simulink model "helicopter_Kalman_4dim"  (R2021b)
settings: Solver=ode45  StartTime=0.0  StopTime=T  RelTol=1e-3
InitFcn:
  | hwinit
values from neighbouring files (symbols this model uses):
  A_lin = [0, 1, 0; K1*cos(alpha_ref), -b, -2*K3*omega_ref; 0, 0, -K4 ]    [observer.m]
  B_lin = [0;0; -K4]    [observer.m]
  C = [1, 0, 0; 0, 0, 1]    [controller_LQR.m]    (also in controller_MPC.m; helicopter_EKF_code.m; observer.m; polish_MPC.m)
  h = 0.01    [Pure_Kalman_check.m]    (also in calibration.m; controller_LQR.m; controller_MPC.m; helicopter_EKF_code.m)
  K = place(A_lin, B_lin, p_new)    [helicopter_EKF_code.m]
  x_ref = sdpvar(n_x, 1)    [MPC_step.m]    (also in controller_LQR.m = [alpha_ref; alpha_dot_ref; omega_ref]/0.9; controller_MPC.m = [alpha_ref; alpha_dot_ref; omega_ref]; helicopter_EKF_code.m = [alpha_ref; alpha_dot_ref; omega_ref]; polish_MPC.m = [alpha_ref; alpha_dot_ref ; omega_ref])
undefined symbols (not defined in the file or in its folder): adingain, adinoffs, Continuous, HeliMexHandle, Time
libraries: ctrlSharedLib x1
settings Model: Creator=fkzhang  LastModifiedBy=lcaric
settings SolverCC: AlgebraicLoopSolver=TrustRegion
settings DataIOCC: LimitDataPoints=on  SaveFormat=Array  ReturnWorkspaceOutputs=off
settings OptimizationCC: BlockReduction=off  BooleanDataType=off  LifeSpan=inf
settings DebuggingCC: SaveWithParameterizedLinksMsg=none  UnderspecifiedInitializationDetection=Classic  MergeDetectMultiDrivingBlocksExec=none  SignalResolutionControl=TryResolveAllWithWarning  AllowSymbolicDim=off  SFUnexpectedBacktrackingDiag=warning  SFNoUnconditionalDefaultTransitionDiag=warning  SFExecutionAtInitializationDiag=none  SFMachineParentedDataDiag=warning  ArithmeticOperatorsInVariantConditions=warning
settings HardwareCC: ProdBitPerPointer=32  ProdBitPerSizeT=32  ProdBitPerPtrDiffT=32  ProdLargestAtomicFloat=None  ProdIntDivRoundTo=Undefined  ProdEndianess=Unspecified  ProdWordSize=32  ProdHWDeviceType=32-bit Generic  TargetUnknown=on
settings ModelReferenceCC: PropagateSignalLabelsOutOfModel=off
settings SFSimCC: SimUseLocalCustomCode=off  CustomCodeUndefinedFunction=UseInterfaceOnly
settings RTWCC: RTWUseLocalCustomCode=off
settings CodeAppCC: StateflowObjectComments=on
settings GRTTargetCC: TargetLangStandard=C89/C90 (ANSI)
settings ConfigComp: CovMetricSettings=dw  CovSaveCumulativeToWorkspaceVar=on  CovSaveSingleToWorkspaceVar=on  CovExternalEMLEnable=off  CovSFcnEnable=off

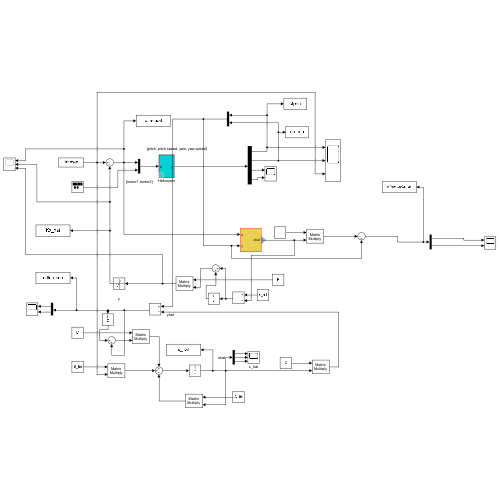
[thumbnail: Simulink's stored preview of the top-level diagram]
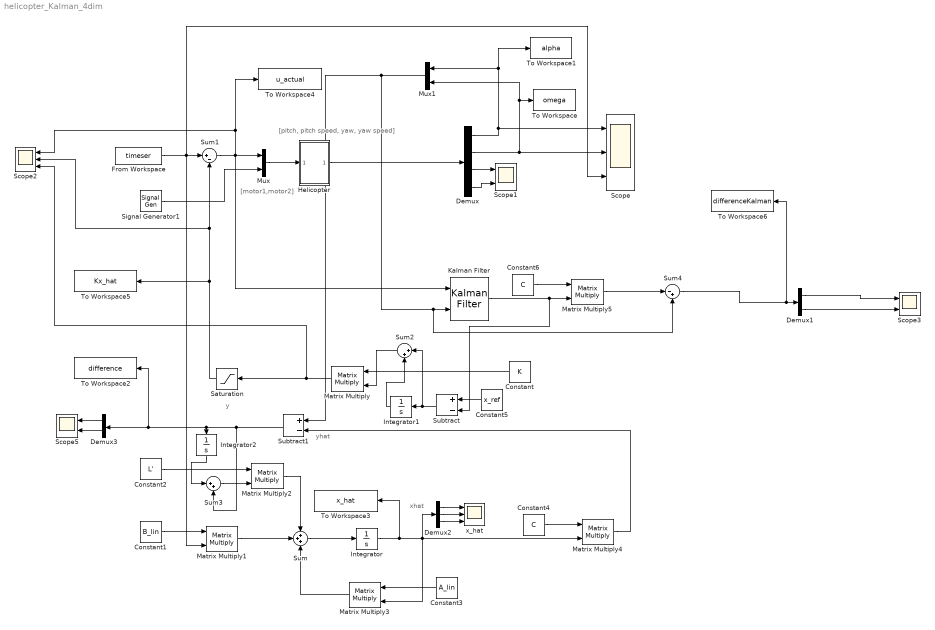
== system helicopter_Kalman_4dim ==
  note: yhat
  note: y
  note: xhat
  note: [pitch, pitch speed, yaw, yaw speed]
  note: [motor1,motor2]
  Constant : Constant  Value=K  VectorParams1D=off
  Constant1 : Constant  Value=B_lin  VectorParams1D=off
  Constant2 : Constant  Value=L'
  Constant3 : Constant  Value=A_lin
  Constant4 : Constant  Value=C
  Constant5 : Constant  Value=x_ref
  Constant6 : Constant  Value=C
  Demux : Demux
  Demux1 : Demux  Outputs=2
  Demux2 : Demux  Outputs=3
  Demux3 : Demux  Outputs=2
  From Workspace : FromWorkspace  VariableName=timeser
  Helicopter : Subsystem  mask{Ts=h}
      mask prompts: Ts "sampletime"
      mask init:
      | sf_heli_init
      mask Display:
      | port_label('input',1,'u');
      | port_label('output',1,'y');
  Integrator : Integrator
  Integrator1 : Integrator
  Integrator2 : Integrator
  Kalman Filter : ctrlSharedLib/Kalman Filter  TimeDomain=Continuous-Time  UseCurrentEstimator=on  ModelSource=LTI State-Space Variable  ModelSourceVariable=minssss  A=A_lin  B=B_lin  C=C  D=[0;0]  NumberOfStates=1  NumberOfInputs=1  NumberOfOutputs=1  InitialEstimateSource=Dialog  X0=[0;0;0;0]  P0=10  UseK=off  UseGH=off  NumberOfProcessNoiseInputs=1  G=1  TimeInvariantG=on  H=0  TimeInvariantH=on  Q=5*eye(3)  TimeInvariantQ=on  R=0.5*eye(2)  TimeInvariantR=on  N=0  TimeInvariantN=on  AddInputPort=on  AddEnablePort=off  OutputEstimatedY=off  OutputP=off  Ts=-1
  Matrix Multiply{,1..5} (6 alike) : Product  Multiplication=Matrix(*)
  Mux : Mux  Inputs=2
  Mux1 : Mux  Inputs=2
  Saturation : Saturate  UpperLimit=1  LowerLimit=-1
  Scope : Scope  NumInputPorts=3
  Scope1 : Scope  NumInputPorts=2
  Scope2 : Scope  NumInputPorts=3
  Scope3 : Scope  NumInputPorts=2
  Scope5 : Scope  NumInputPorts=2
  Signal Generator1 : SignalGenerator  WaveForm=square  Amplitude=0  Frequency=1/20
  Subtract : Sum  Inputs=+-
  Subtract1 : Sum  Inputs=+-
  Sum : Sum  Inputs=+++
  Sum1 : Sum  Inputs=|+-
  Sum2 : Sum  Inputs=|++
  Sum3 : Sum  Inputs=|++
  Sum4 : Sum  Inputs=|-+
  To Workspace : ToWorkspace  VariableName=omega  SaveFormat=Timeseries  SampleTime=-1
  To Workspace1 : ToWorkspace  VariableName=alpha  SaveFormat=Timeseries  SampleTime=-1
  To Workspace2 : ToWorkspace  VariableName=difference  SaveFormat=Timeseries  SampleTime=-1
  To Workspace3 : ToWorkspace  VariableName=x_hat  SaveFormat=Timeseries  SampleTime=-1
  To Workspace4 : ToWorkspace  VariableName=u_actual  SaveFormat=Timeseries  SampleTime=-1
  To Workspace5 : ToWorkspace  VariableName=Kx_hat  SaveFormat=Timeseries  SampleTime=-1
  To Workspace6 : ToWorkspace  VariableName=differenceKalman  SaveFormat=Timeseries  SampleTime=-1
  x_hat : Scope  NumInputPorts=3
  wires:
  Mux/1 -> Helicopter/1(In1)
  Signal Generator1/1 -> Mux/2
  Demux/2 -> Scope/2, To Workspace/1, Mux1/2
  Demux/3 -> Scope1/1
  Demux/4 -> Scope1/2
  From Workspace/1 -> Sum1/1, Matrix Multiply1/2, Scope/3
  Demux/1 -> To Workspace1/1, Mux1/1, Scope/1
  Mux1/1 -> Sum4/2, Kalman Filter/2, Subtract1/1
  Helicopter/1(Out1) -> Demux/1
  Matrix Multiply1/1 -> Sum/2
  Matrix Multiply2/1 -> Sum/1
  Sum/1 -> Integrator/1
  Matrix Multiply3/1 -> Sum/3
  Integrator/1 -> To Workspace3/1, Matrix Multiply3/2, Matrix Multiply4/2, Demux2/1
  Demux2/2 -> x_hat/2
  Demux2/3 -> x_hat/3
  Demux2/1 -> x_hat/1
  Matrix Multiply4/1 -> Subtract1/2
  Demux3/2 -> Scope5/2
  Demux3/1 -> Scope5/1
  Constant1/1 -> Matrix Multiply1/1
  Constant2/1 -> Matrix Multiply2/1
  Constant4/1 -> Matrix Multiply4/1
  Constant3/1 -> Matrix Multiply3/1
  Sum1/1 -> Kalman Filter/1, To Workspace4/1, Scope2/1, Mux/1
  Constant/1 -> Matrix Multiply/1
  Saturation/1 -> To Workspace5/1, Scope2/2, Sum1/2
  Matrix Multiply/1 -> Saturation/1, Scope2/3
  Constant5/1 -> Subtract/1
  Subtract/1 -> Sum2/1, Integrator1/1
  Integrator1/1 -> Sum2/2
  Sum2/1 -> Matrix Multiply/2
  Subtract1/1 -> To Workspace2/1, Demux3/1, Integrator2/1, Sum3/2
  Demux1/2 -> Scope3/2
  Demux1/1 -> Scope3/1
  Constant6/1 -> Matrix Multiply5/1
  Kalman Filter/1 -> Subtract/2, Matrix Multiply5/2
  Matrix Multiply5/1 -> Sum4/1
  Sum4/1 -> To Workspace6/1, Demux1/1
  Integrator2/1 -> Sum3/1
  Sum3/1 -> Matrix Multiply2/2

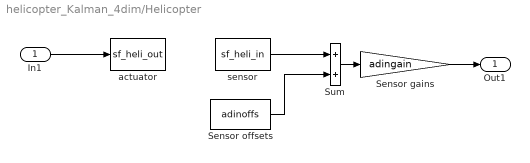
== system helicopter_Kalman_4dim/Helicopter ==
  In1 : Inport
  Sensor gains : Gain  Gain=adingain
  Sensor offsets : Constant  Value=adinoffs
  Sum : Sum
  actuator : M-S-Function  FunctionName=sf_heli_out  Parameters=HeliMexHandle,Ts
  sensor : M-S-Function  FunctionName=sf_heli_in  Parameters=HeliMexHandle
  Out1 : Outport  VectorParamsAs1DForOutWhenUnconnected=off
  wires:
  sensor/1 -> Sum/1
  In1/1 -> actuator/1
  Sensor offsets/1 -> Sum/2
  Sum/1 -> Sensor gains/1
  Sensor gains/1 -> Out1/1
